simulink model "Sensor_Reading_Filter"  (R2021b)
settings: Solver=VariableStepAuto  StartTime=0.0  StopTime=10  RelTol=1e-3
undefined symbols (not defined in the file): sigbuilder_block
settings Model: NumberOfSteps=4  Creator=t  LastModifiedBy=t

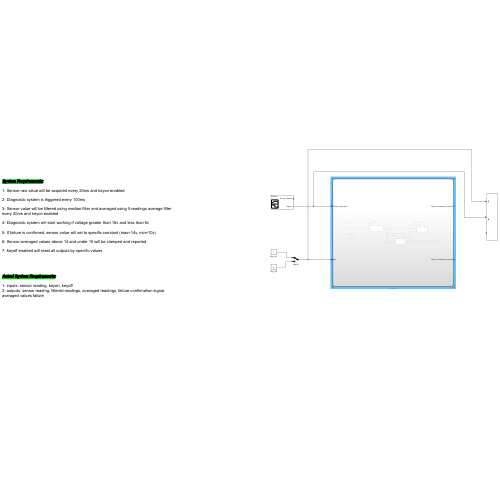
[thumbnail: Simulink's stored preview of the top-level diagram]
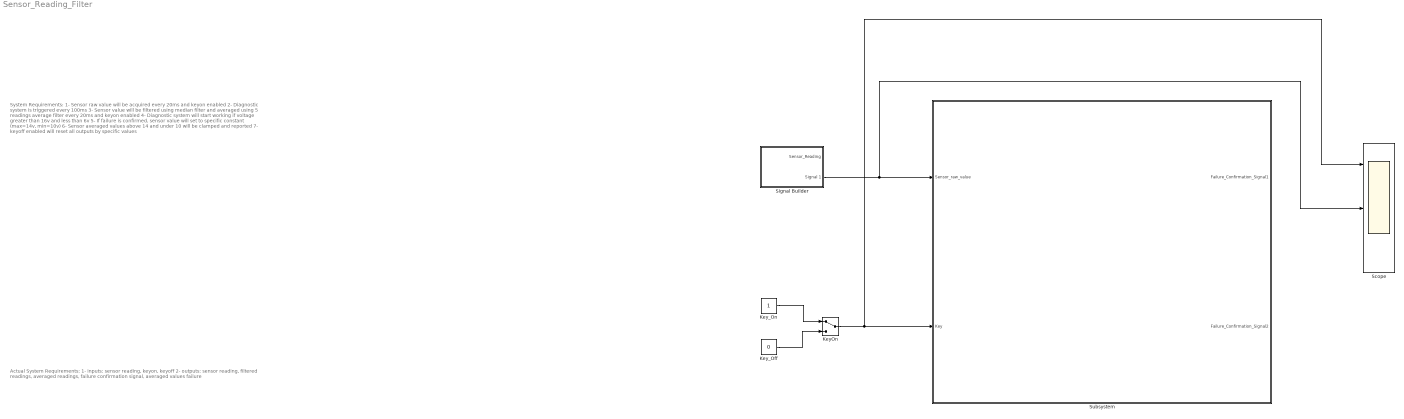
== system Sensor_Reading_Filter ==
  note: System Requirements:
      |
      | 1- Sensor raw value will be acquired every 20ms and keyon enabled
      |
      | 2- Diagnostic system is triggered every 100ms
      |
      | 3- Sensor value will be filtered using median filter and averaged using 5 readings average filter every 20ms and keyon enabled
      |
      | 4- Diagnostic system will start working if voltage greater than 16v and less than 6v
      |
      | 5- If failure is confirmed, sensor value will set to specific constant (max=14v, min=10v)
      |
      | 6- Sensor averaged values above 14 and under 10 will be clamped and reported
      |
      | 7- keyoff enabled will reset all outputs by specific values
  note: Actual System Requirements:
      |
      | 1- inputs: sensor reading, keyon, keyoff
      | 2- outputs: sensor reading, filtered readings, averaged readings, failure confirmation signal, averaged values failure
  KeyOn : ManualSwitch
  Key_Off : Constant  Value=0
  Key_On : Constant
  Scope : Scope  NumInputPorts=3
  Signal Builder : Subsystem  Tag=STV Subsys  LoadFcn=sigbuilder_block('load');  StartFcn=sigbuilder_block('start');  StopFcn=sigbuilder_block('stop');  ClipboardFcn=sigbuilder_block('clipboard');  mask(Sigbuilder block){tuvar=[0:10]}
      mask help: Simulink:masks:SigbuilderBlock_MD
      mask init:
      | if ~strcmp(get_param(bdroot(gcbh),'SimulationStatus'),'stopped') tuvar = sigbuilder_block('maskInit'); end
      settings: CopyFcn=sigbuilder_block('copy');  DeleteFcn=sigbuilder_block('delete');  ModelCloseFcn=sigbuilder_block('modelClose');  PreSaveFcn=sigbuilder_block('preSave');  PauseFcn=sigbuilder_block('pause');  ContinueFcn=sigbuilder_block('continue');  NameChangeFcn=sigbuilder_block('namechange');  OpenFcn=sigbuilder_block('open',[5.4 30 1141.2 522.6 ]);  CloseFcn=sigbuilder_block('close');
      mask Display: plot(0, 0, 100, 100,[2, 2, 32, 32, 2], [68, 8, 8, 68, 68],[32, 2], [38, 38], [32, 19, 2],[53, 60, 44], [32, 17, 17, 2],[16, 16, 31, 31]);txt = getActiveGroup(gcbh);text(2, 100, txt,'verticalAlignment', 'top');
  Subsystem : Subsystem
  wires:
  KeyOn/1 -> Subsystem/2(Key), Scope/1
  Key_On/1 -> KeyOn/1
  Key_Off/1 -> KeyOn/2
  Signal Builder/2(Signal 1) -> Scope/2, Subsystem/1(Sensor_raw_value)

== system Sensor_Reading_Filter/Signal Builder ==
  Demux : Demux  Tag=STV Demux  Outputs=2
      settings: DisplayOption=none
  FromWs : FromWorkspace  Tag=STV FromWs  VariableName=tuvar
      SigBuilderData=|
      | common.afterFinalStr = 'Extrapolate'
      | common.sampleTime = 0
      | dataSet.timeRange = [0 10]
      | dataSet.name = 'Group 1'
      | sbobj.Groups.Name = 'Group 1'
      | sbobj.Groups.Signals(1).Name = 'Sensor_Reading'
      | sbobj.Groups.Signals(1).XData = [0 0.125 0.25 0.375 0.5 0.625 0.75 0.875 1 1.125 1.25 1.375 1.5 1.625 1.75 1.875 2 2.125 2.25 2.375 2.5 2.625 2.75 2.875 3 3.125 3.25 3.375 3.5 3.625 3.75 3.875 4 4.125 4.25 4.375 4.5 4.625 4.75 4.875 5 5.125 5.25 5.375 5.5 5.625 5.75 5.875 6 6.125 6.25 6.375 6.5 6.625 6.75 6.875 7 7.125 7.25 7.375 7.5 7.625 7.75 7.875 8 8.125 8.25 8.375 8.5 8.625 8.75 8.875 9 9.125 9.25 9.375 9.5 9.625 9.75 9.875 10]
      | sbobj.Groups.Signals(1).YData = [10 15.6568542495 18 15.6568542495 10 4.34314575051 2 4.34314575051 10 15.6568542495 18 15.6568542495 10 4.34314575051 2 4.34314575051 10 15.6568542495 18 15.6568542495 10 4.34314575051 2 4.34314575051 10 15.6568542495 18 15.6568542495 10 4.34314575051 2 4.34314575051 10 15.6568542495 18 15.6568542495 10 4.34314575051 2 4.34314575051 10 15.6568542495 18 15.6568542495 10 4.34314575051 2 4.34314575051 10 15.6568542495 18 15.6568542495 10 4.34314575051 2 4.34314575051 10 15.6568542495 18 15.6568542495 10 4.34314575051 2 4.34314575051 10 15.6568542495 18 15.6568542495 10 4.34314575051 2 4.34314575051 10 15.6568542495 18 15.6568542495 10 4.34314575051 2 4.34314575051 10]
      | sbobj.Groups.Signals(2).Name = 'Signal 1'
      | sbobj.Groups.Signals(2).XData = [0 4.44 10]
      | sbobj.Groups.Signals(2).YData = [18 18 18]
  Sensor_Reading : Outport  Tag=STV Outport
  Signal 1 : Outport  Tag=STV Outport  Port=2
  wires:
  FromWs/1 -> Demux/1
  Demux/1 -> Sensor_Reading/1
  Demux/2 -> Signal 1/1

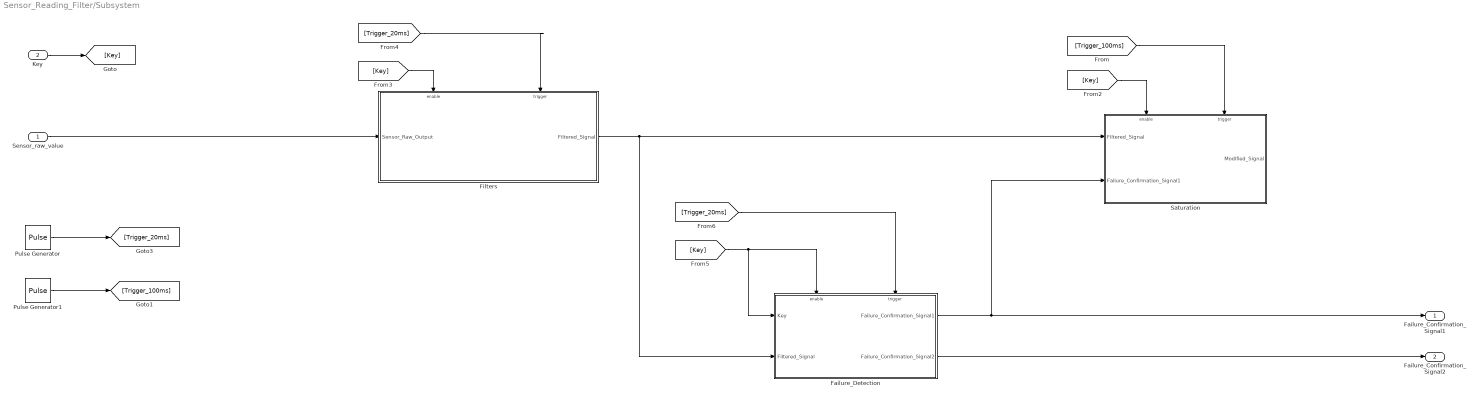
== system Sensor_Reading_Filter/Subsystem ==
  Sensor_raw_value : Inport
  Key : Inport  Port=2
  Failure_Detection : Subsystem
  Filters : Subsystem
  Pulse Generator : DiscretePulseGenerator  SampleTime=0.1
  Pulse Generator1 : DiscretePulseGenerator  SampleTime=0.5
  Saturation : Subsystem
  Failure_Confirmation_Signal1 : Outport
  Failure_Confirmation_Signal2 : Outport  Port=2
  wires:
  Key/1 -> [Key]
  Pulse Generator/1 -> [Trigger_20ms]
  Pulse Generator1/1 -> [Trigger_100ms]
  [Key] -> Filters/Enable
  [Trigger_20ms] -> Filters/Trigger
  [Key] -> Saturation/Enable
  [Trigger_100ms] -> Saturation/Trigger
  Filters/1(Filtered_Signal) -> Failure_Detection/2(Filtered_Signal), Saturation/1(Filtered_Signal)
  [Key] -> Failure_Detection/1(Key), Failure_Detection/Enable
  [Trigger_20ms] -> Failure_Detection/Trigger
  Failure_Detection/1(Failure_Confirmation_Signal1) -> Saturation/2(Failure_Confirmation_Signal1), Failure_Confirmation_Signal1/1
  Sensor_raw_value/1 -> Filters/1(Sensor_Raw_Output)
  Failure_Detection/2(Failure_Confirmation_Signal2) -> Failure_Confirmation_Signal2/1

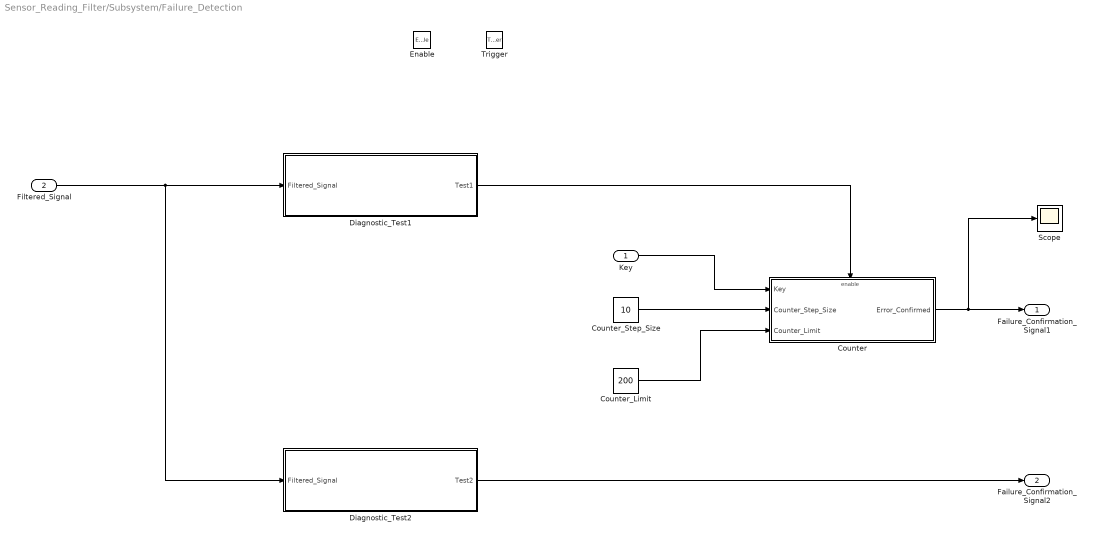
== system Sensor_Reading_Filter/Subsystem/Failure_Detection ==
  Key : Inport
  Filtered_Signal : Inport  Port=2
  Enable : EnablePort
  Trigger : TriggerPort  VariantControl=(inherit)  PortDimensions=1
  Counter : Subsystem
  Counter_Limit : Constant  Value=200
  Counter_Step_Size : Constant  Value=10
  Diagnostic_Test1 : Subsystem
  Diagnostic_Test2 : Subsystem
  Scope : Scope
  Failure_Confirmation_Signal1 : Outport
  Failure_Confirmation_Signal2 : Outport  Port=2
  wires:
  Filtered_Signal/1 -> Diagnostic_Test2/1(Filtered_Signal), Diagnostic_Test1/1(Filtered_Signal)
  Diagnostic_Test1/1(Test1) -> Counter/Enable
  Counter_Step_Size/1 -> Counter/2(Counter_Step_Size)
  Counter_Limit/1 -> Counter/3(Counter_Limit)
  Counter/1(Error_Confirmed) -> Scope/1, Failure_Confirmation_Signal1/1
  Diagnostic_Test2/1(Test2) -> Failure_Confirmation_Signal2/1
  Key/1 -> Counter/1(Key)

== system Sensor_Reading_Filter/Subsystem/Filters ==
  Sensor_Raw_Output : Inport
  Enable : EnablePort
  Trigger : TriggerPort  VariantControl=(inherit)  PortDimensions=1
  Sesnsor_Median_Filter : Subsystem  TreatAsAtomicUnit=on
  Sesnsor_Median_Filter1 : Subsystem  TreatAsAtomicUnit=on
  Filtered_Signal : Outport
  wires:
  Sensor_Raw_Output/1 -> Sesnsor_Median_Filter/1(Sensor_Raw_Output)
  Sesnsor_Median_Filter/1(Median_Filtered_Signal) -> Sesnsor_Median_Filter1/1(Median_Filtered_Input)
  Sesnsor_Median_Filter1/1(Averaged_Output_Signal) -> Filtered_Signal/1

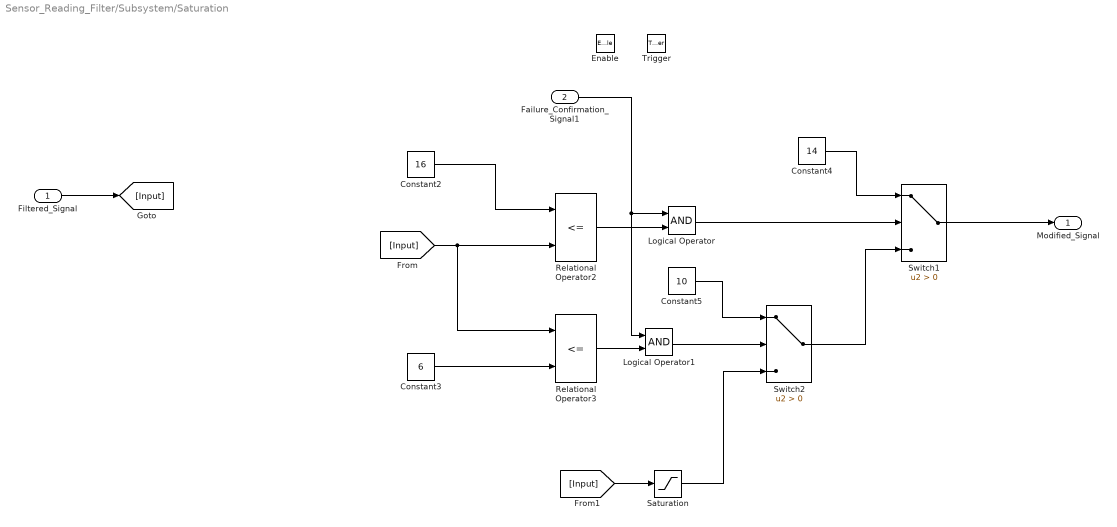
== system Sensor_Reading_Filter/Subsystem/Saturation ==
  Filtered_Signal : Inport
  Failure_Confirmation_Signal1 : Inport  Port=2
  Enable : EnablePort
  Trigger : TriggerPort  VariantControl=(inherit)  PortDimensions=1
  Constant2 : Constant  Value=16
  Constant3 : Constant  Value=6
  Constant4 : Constant  Value=14
  Constant5 : Constant  Value=10
  Logical Operator : Logic  AllPortsSameDT=off  OutDataTypeStr=boolean
  Logical Operator1 : Logic  AllPortsSameDT=off  OutDataTypeStr=boolean
  Relational Operator2 : RelationalOperator  Operator=<=  OutDataTypeStr=boolean  RndMeth=Simplest
  Relational Operator3 : RelationalOperator  Operator=<=  OutDataTypeStr=boolean  RndMeth=Simplest
  Saturation : Saturate  UpperLimit=14  LowerLimit=10
  Switch1 : Switch  Criteria=u2 > Threshold
  Switch2 : Switch  Criteria=u2 > Threshold
  Modified_Signal : Outport
  wires:
  Filtered_Signal/1 -> [Input]
  Constant3/1 -> Relational Operator3/2
  Constant5/1 -> Switch2/1
  [Input] -> Relational Operator3/1, Relational Operator2/2
  Switch2/1 -> Switch1/3
  Constant4/1 -> Switch1/1
  Constant2/1 -> Relational Operator2/1
  [Input] -> Saturation/1
  Switch1/1 -> Modified_Signal/1
  Relational Operator2/1 -> Logical Operator/2
  Logical Operator/1 -> Switch1/2
  Failure_Confirmation_Signal1/1 -> Logical Operator/1, Logical Operator1/1
  Relational Operator3/1 -> Logical Operator1/2
  Logical Operator1/1 -> Switch2/2
  Saturation/1 -> Switch2/3

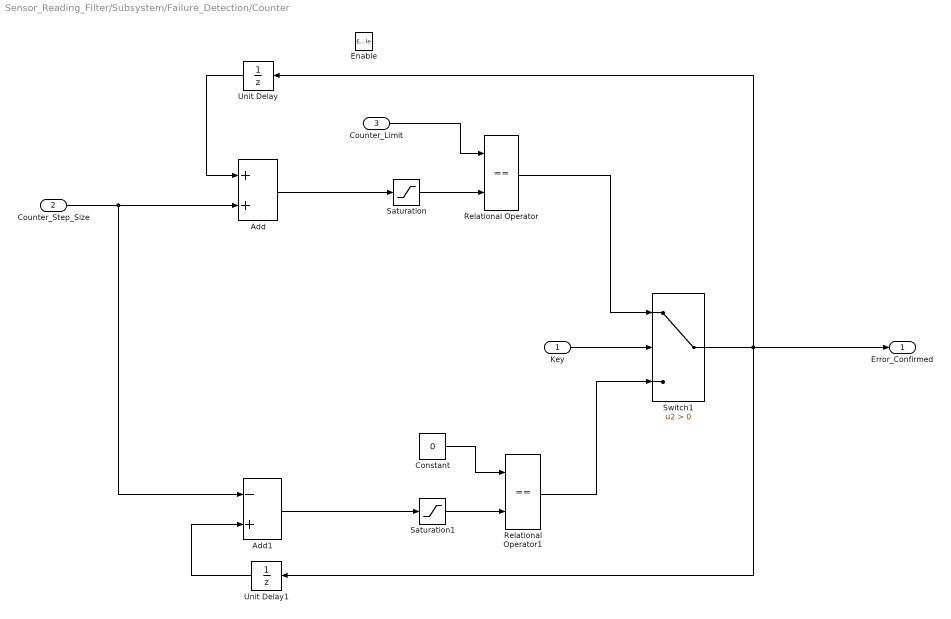
== system Sensor_Reading_Filter/Subsystem/Failure_Detection/Counter ==
  Key : Inport
  Counter_Step_Size : Inport  Port=2
  Counter_Limit : Inport  Port=3
  Enable : EnablePort
  Add : Sum
  Add1 : Sum  Inputs=-+
  Constant : Constant  Value=0
  Relational Operator : RelationalOperator  Operator===  OutDataTypeStr=boolean  RndMeth=Simplest
  Relational Operator1 : RelationalOperator  Operator===  OutDataTypeStr=boolean  RndMeth=Simplest
  Saturation : Saturate  UpperLimit=100  LowerLimit=0
  Saturation1 : Saturate  UpperLimit=100  LowerLimit=0
  Switch1 : Switch  Criteria=u2 > Threshold
  Unit Delay : UnitDelay  SampleTime=-1  HasFrameUpgradeWarning=on
  Unit Delay1 : UnitDelay  SampleTime=-1  HasFrameUpgradeWarning=on
  Error_Confirmed : Outport
  wires:
  Add/1 -> Saturation/1
  Counter_Limit/1 -> Relational Operator/1
  Saturation/1 -> Relational Operator/2
  Unit Delay/1 -> Add/1
  Relational Operator/1 -> Switch1/1
  Key/1 -> Switch1/2
  Unit Delay1/1 -> Add1/2
  Add1/1 -> Saturation1/1
  Counter_Step_Size/1 -> Add/2, Add1/1
  Switch1/1 -> Unit Delay/1, Unit Delay1/1, Error_Confirmed/1
  Saturation1/1 -> Relational Operator1/2
  Relational Operator1/1 -> Switch1/3
  Constant/1 -> Relational Operator1/1

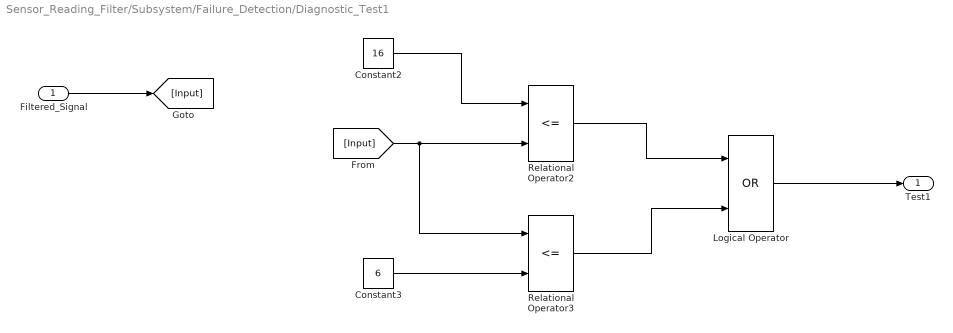
== system Sensor_Reading_Filter/Subsystem/Failure_Detection/Diagnostic_Test1 ==
  Filtered_Signal : Inport
  Constant2 : Constant  Value=16
  Constant3 : Constant  Value=6
  Logical Operator : Logic  Operator=OR  AllPortsSameDT=off  OutDataTypeStr=boolean
  Relational Operator2 : RelationalOperator  Operator=<=  OutDataTypeStr=boolean  RndMeth=Simplest
  Relational Operator3 : RelationalOperator  Operator=<=  OutDataTypeStr=boolean  RndMeth=Simplest
  Test1 : Outport
  wires:
  Constant3/1 -> Relational Operator3/2
  [Input] -> Relational Operator3/1, Relational Operator2/2
  Constant2/1 -> Relational Operator2/1
  Filtered_Signal/1 -> [Input]
  Relational Operator2/1 -> Logical Operator/1
  Relational Operator3/1 -> Logical Operator/2
  Logical Operator/1 -> Test1/1

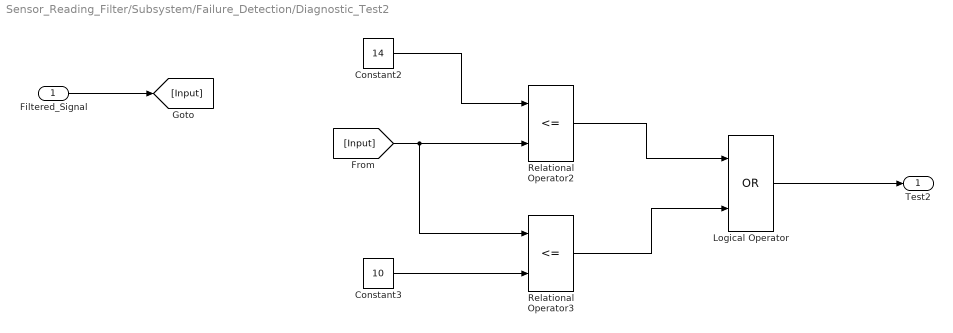
== system Sensor_Reading_Filter/Subsystem/Failure_Detection/Diagnostic_Test2 ==
  Filtered_Signal : Inport
  Constant2 : Constant  Value=14
  Constant3 : Constant  Value=10
  Logical Operator : Logic  Operator=OR  AllPortsSameDT=off  OutDataTypeStr=boolean
  Relational Operator2 : RelationalOperator  Operator=<=  OutDataTypeStr=boolean  RndMeth=Simplest
  Relational Operator3 : RelationalOperator  Operator=<=  OutDataTypeStr=boolean  RndMeth=Simplest
  Test2 : Outport
  wires:
  Logical Operator/1 -> Test2/1
  Relational Operator3/1 -> Logical Operator/2
  Relational Operator2/1 -> Logical Operator/1
  Filtered_Signal/1 -> [Input]
  Constant2/1 -> Relational Operator2/1
  [Input] -> Relational Operator2/2, Relational Operator3/1
  Constant3/1 -> Relational Operator3/2

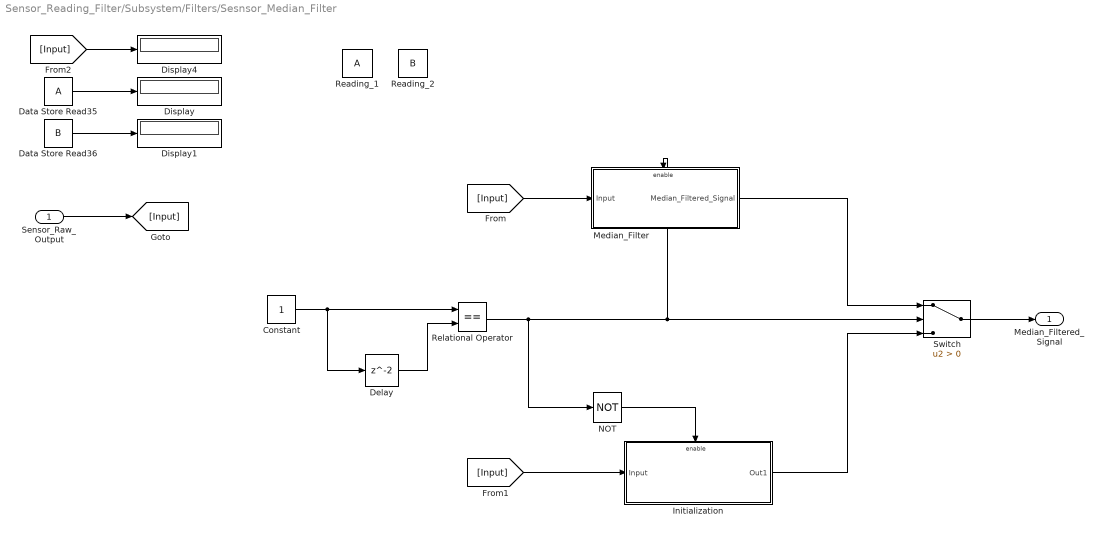
== system Sensor_Reading_Filter/Subsystem/Filters/Sesnsor_Median_Filter ==
  Sensor_Raw_Output : Inport
  Constant : Constant
  Data Store Read35 : DataStoreRead  IndexOptions=Index vector (dialog)  Indices=1  OutputSizes=1
  Data Store Read36 : DataStoreRead  DataStoreName=B  IndexOptions=Index vector (dialog)  Indices=1  OutputSizes=1
  Delay : Delay
  Display : Display
  Display1 : Display
  Display4 : Display
  Initialization : Subsystem
  Median_Filter : Subsystem
  NOT : Logic  Operator=NOT  IconShape=distinctive  AllPortsSameDT=off  OutDataTypeStr=boolean
  Reading_1 : DataStoreMemory  ReadBeforeWriteMsg=warning  WriteAfterWriteMsg=warning  WriteAfterReadMsg=warning  ShowAdditionalParam=off
  Reading_2 : DataStoreMemory  DataStoreName=B  ReadBeforeWriteMsg=warning  WriteAfterWriteMsg=warning  WriteAfterReadMsg=warning  ShowAdditionalParam=off
  Relational Operator : RelationalOperator  Operator===  OutDataTypeStr=boolean  RndMeth=Simplest
  Switch : Switch  Criteria=u2 > Threshold
  Median_Filtered_Signal : Outport
  wires:
  Data Store Read35/1 -> Display/1
  Data Store Read36/1 -> Display1/1
  Constant/1 -> Delay/1, Relational Operator/1
  Delay/1 -> Relational Operator/2
  Relational Operator/1 -> NOT/1, Median_Filter/Enable, Switch/2
  NOT/1 -> Initialization/Enable
  Initialization/1(Out1) -> Switch/3
  Median_Filter/1(Median_Filtered_Signal) -> Switch/1
  Sensor_Raw_Output/1 -> [Input]
  [Input] -> Median_Filter/1(Input)
  [Input] -> Initialization/1(Input)
  [Input] -> Display4/1
  Switch/1 -> Median_Filtered_Signal/1

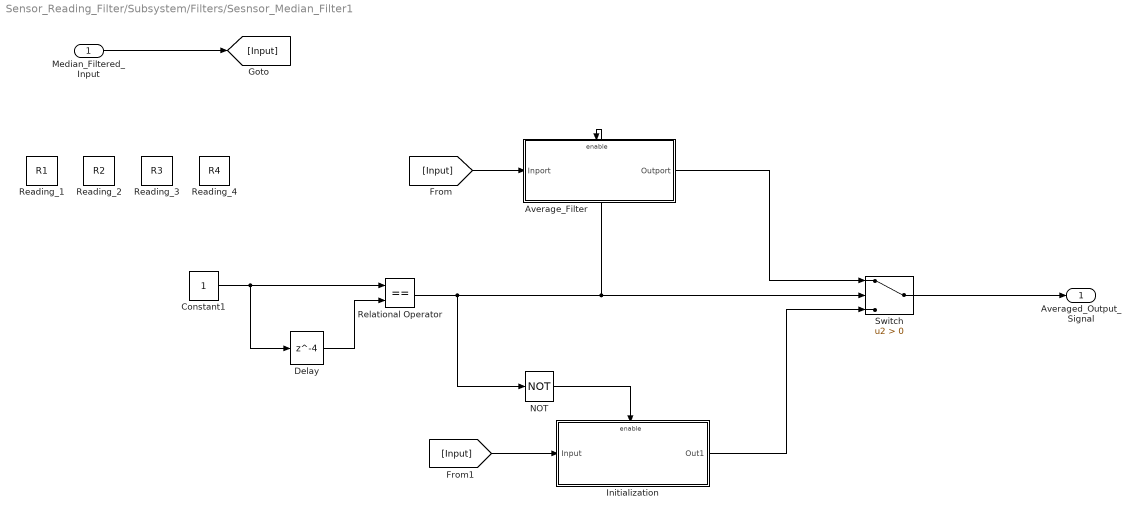
== system Sensor_Reading_Filter/Subsystem/Filters/Sesnsor_Median_Filter1 ==
  Median_Filtered_Input : Inport
  Average_Filter : Subsystem
  Constant1 : Constant
  Delay : Delay  DelayLength=4
  Initialization : Subsystem
  NOT : Logic  Operator=NOT  IconShape=distinctive  AllPortsSameDT=off  OutDataTypeStr=boolean
  Reading_1 : DataStoreMemory  DataStoreName=R1  ReadBeforeWriteMsg=warning  WriteAfterWriteMsg=warning  WriteAfterReadMsg=warning  ShowAdditionalParam=off
  Reading_2 : DataStoreMemory  DataStoreName=R2  ReadBeforeWriteMsg=warning  WriteAfterWriteMsg=warning  WriteAfterReadMsg=warning  ShowAdditionalParam=off
  Reading_3 : DataStoreMemory  DataStoreName=R3  ReadBeforeWriteMsg=warning  WriteAfterWriteMsg=warning  WriteAfterReadMsg=warning  ShowAdditionalParam=off
  Reading_4 : DataStoreMemory  DataStoreName=R4  ReadBeforeWriteMsg=warning  WriteAfterWriteMsg=warning  WriteAfterReadMsg=warning  ShowAdditionalParam=off
  Relational Operator : RelationalOperator  Operator===  OutDataTypeStr=boolean  RndMeth=Simplest
  Switch : Switch  Criteria=u2 > Threshold
  Averaged_Output_Signal : Outport
  wires:
  Median_Filtered_Input/1 -> [Input]
  Switch/1 -> Averaged_Output_Signal/1
  Delay/1 -> Relational Operator/2
  Initialization/1(Out1) -> Switch/3
  NOT/1 -> Initialization/Enable
  Relational Operator/1 -> NOT/1, Average_Filter/Enable, Switch/2
  Constant1/1 -> Delay/1, Relational Operator/1
  [Input] -> Average_Filter/1(Inport)
  [Input] -> Initialization/1(Input)
  Average_Filter/1(Outport) -> Switch/1

== system Sensor_Reading_Filter/Subsystem/Filters/Sesnsor_Median_Filter/Initialization ==
  Input : Inport
  Enable : EnablePort
  Data Store Write : DataStoreWrite  IndexOptions=Index vector (dialog)  Indices=1  OutputSizes=1
  Data Store Write1 : DataStoreWrite  DataStoreName=B  IndexOptions=Index vector (dialog)  Indices=1  OutputSizes=1
  Unit Delay1 : UnitDelay  SampleTime=-1  HasFrameUpgradeWarning=on
  Out1 : Outport
  wires:
  Unit Delay1/1 -> Data Store Write1/1
  Input/1 -> Data Store Write/1, Out1/1, Unit Delay1/1

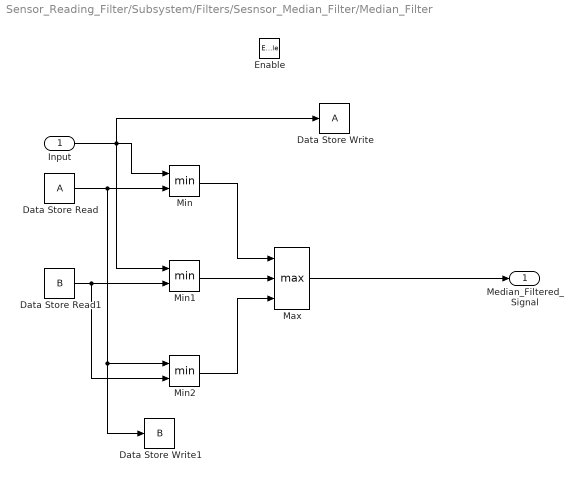
== system Sensor_Reading_Filter/Subsystem/Filters/Sesnsor_Median_Filter/Median_Filter ==
  Input : Inport
  Enable : EnablePort
  Data Store Read : DataStoreRead  IndexOptions=Index vector (dialog)  Indices=1  OutputSizes=1
  Data Store Read1 : DataStoreRead  DataStoreName=B  IndexOptions=Index vector (dialog)  Indices=1  OutputSizes=1
  Data Store Write : DataStoreWrite  IndexOptions=Index vector (dialog)  Indices=1  OutputSizes=1
  Data Store Write1 : DataStoreWrite  DataStoreName=B  IndexOptions=Index vector (dialog)  Indices=1  OutputSizes=1
  Max : MinMax  Function=max  Inputs=3
  Min : MinMax  Inputs=2
  Min1 : MinMax  Inputs=2
  Min2 : MinMax  Inputs=2
  Median_Filtered_Signal : Outport
  wires:
  Input/1 -> Data Store Write/1, Min1/1, Min/1
  Data Store Read/1 -> Data Store Write1/1, Min2/1, Min/2
  Data Store Read1/1 -> Min2/2, Min1/2
  Min1/1 -> Max/2
  Min/1 -> Max/1
  Min2/1 -> Max/3
  Max/1 -> Median_Filtered_Signal/1

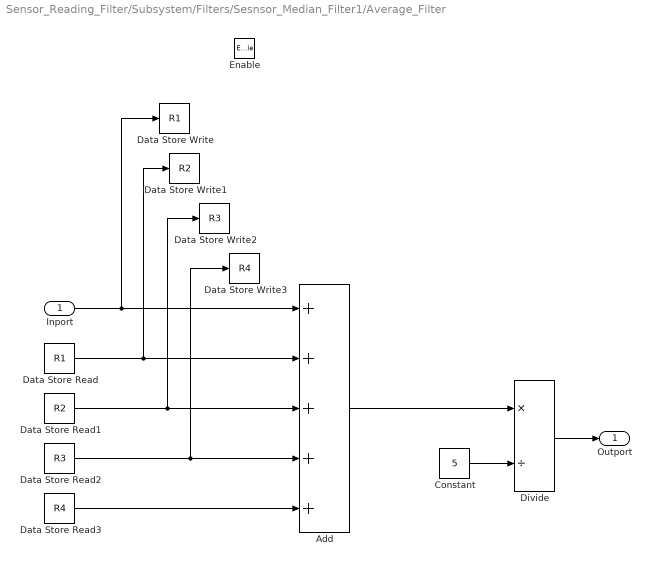
== system Sensor_Reading_Filter/Subsystem/Filters/Sesnsor_Median_Filter1/Average_Filter ==
  Inport : Inport
  Enable : EnablePort
  Add : Sum  Inputs=+++++
  Constant : Constant  Value=5
  Data Store Read : DataStoreRead  DataStoreName=R1  IndexOptions=Index vector (dialog)  Indices=1  OutputSizes=1
  Data Store Read1 : DataStoreRead  DataStoreName=R2  IndexOptions=Index vector (dialog)  Indices=1  OutputSizes=1
  Data Store Read2 : DataStoreRead  DataStoreName=R3  IndexOptions=Index vector (dialog)  Indices=1  OutputSizes=1
  Data Store Read3 : DataStoreRead  DataStoreName=R4  IndexOptions=Index vector (dialog)  Indices=1  OutputSizes=1
  Data Store Write : DataStoreWrite  DataStoreName=R1  IndexOptions=Index vector (dialog)  Indices=1  OutputSizes=1
  Data Store Write1 : DataStoreWrite  DataStoreName=R2  IndexOptions=Index vector (dialog)  Indices=1  OutputSizes=1
  Data Store Write2 : DataStoreWrite  DataStoreName=R3  IndexOptions=Index vector (dialog)  Indices=1  OutputSizes=1
  Data Store Write3 : DataStoreWrite  DataStoreName=R4  IndexOptions=Index vector (dialog)  Indices=1  OutputSizes=1
  Divide : Product  Inputs=*/
  Outport : Outport
  wires:
  Data Store Read2/1 -> Add/4, Data Store Write3/1
  Data Store Read/1 -> Add/2, Data Store Write1/1
  Divide/1 -> Outport/1
  Data Store Read1/1 -> Add/3, Data Store Write2/1
  Inport/1 -> Add/1, Data Store Write/1
  Add/1 -> Divide/1
  Data Store Read3/1 -> Add/5
  Constant/1 -> Divide/2

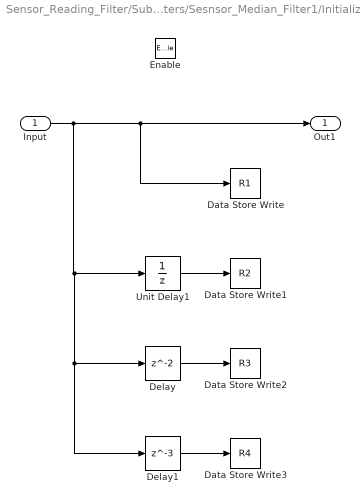
== system Sensor_Reading_Filter/Subsystem/Filters/Sesnsor_Median_Filter1/Initialization ==
  Input : Inport
  Enable : EnablePort
  Data Store Write : DataStoreWrite  DataStoreName=R1  IndexOptions=Index vector (dialog)  Indices=1  OutputSizes=1
  Data Store Write1 : DataStoreWrite  DataStoreName=R2  IndexOptions=Index vector (dialog)  Indices=1  OutputSizes=1
  Data Store Write2 : DataStoreWrite  DataStoreName=R3  IndexOptions=Index vector (dialog)  Indices=1  OutputSizes=1
  Data Store Write3 : DataStoreWrite  DataStoreName=R4  IndexOptions=Index vector (dialog)  Indices=1  OutputSizes=1
  Delay : Delay
  Delay1 : Delay  DelayLength=3
  Unit Delay1 : UnitDelay  SampleTime=-1  HasFrameUpgradeWarning=on
  Out1 : Outport
  wires:
  Unit Delay1/1 -> Data Store Write1/1
  Input/1 -> Data Store Write/1, Out1/1, Delay/1, Delay1/1, Unit Delay1/1
  Delay1/1 -> Data Store Write3/1
  Delay/1 -> Data Store Write2/1
